simulink model "NMPC_MD_gaslift"  (R2023a)
settings: Solver=ode15s  StartTime=0.0  StopTime=par.simulation_time  FixedStep=par.sample_time  RelTol=1e-3
values from neighbouring files (symbols this model uses):
  par = function_parameters_NMPC_MD_gaslift    [main_NMPC_MD_gaslift.m]
  u0 = [par.Qginj0; par.pres]    [main_NMPC_MD_gaslift.m]
  x0 = [par.mg0; par.ml0; 0]    [main_NMPC_MD_gaslift.m]
libraries: sharedTrackingLibrary x1, mpclib x1
settings Model: Creator=aslik  LastModifiedBy=aslik
settings DataIOCC: ReturnWorkspaceOutputs=off  DatasetSignalFormat=timetable

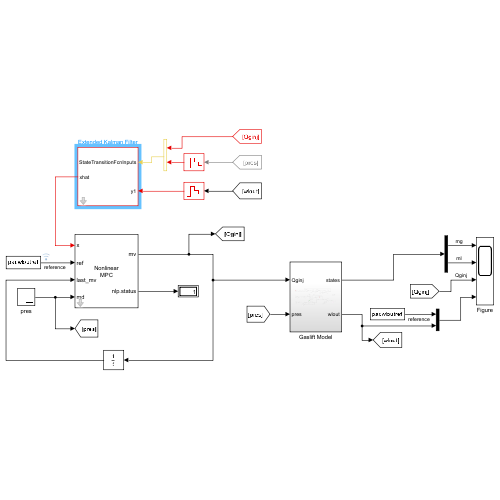
[thumbnail: Simulink's stored preview of the top-level diagram]
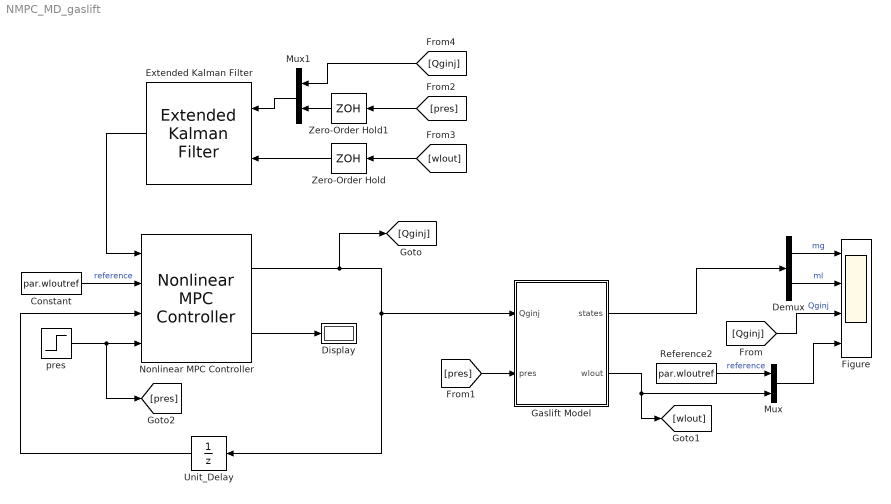
== system NMPC_MD_gaslift ==
  Constant : Constant  Value=par.wloutref  OutDataTypeStr=double  SampleTime=0
  Demux : Demux  Outputs=2
  Display : Display
  Extended Kalman Filter : sharedTrackingLibrary/Extended Kalman Filter  StateTransitionFcn=function_state_discrete_MD_gaslift  HasStateTransitionJacobianFcn=off  HasAdditiveProcessNoise=Additive  ProcessNoise=[2.213446776634616e-09,-7.436473103160610e-07,0;-7.436473103160610e-07,2.499957800870366e-04,0;0,0,0.002500000000000]  HasTimeVaryingProcessNoise=off  HasStateTransitionFcnExtraArgument=1  InitialState=x0  InitialStateCovariance=[2.213446776634616e-09,-7.436473103160610e-07,0;-7.436473103160610e-07,2.499957800870366e-04,0;0,0,0.002500000000000]  MeasurementFcn1=function_measurement_MD_gaslift  HasMeasurementJacobianFcn1=off  HasMeasurementEnablePort1=off  HasAdditiveMeasurementNoise1=Additive  MeasurementNoise1=1  HasTimeVaryingMeasurementNoise1=off  HasMeasurementFcnExtraArgument1=0  HasMeasurementWrapping1=off  MeasurementFcn2=myMeasurementFcn  HasMeasurementJacobianFcn2=off  HasMeasurementEnablePort2=off  HasAdditiveMeasurementNoise2=Additive  MeasurementNoise2=1  HasTimeVaryingMeasurementNoise2=off  HasMeasurementFcnExtraArgument2=0  HasMeasurementWrapping2=off  MeasurementFcn3=myMeasurementFcn  HasMeasurementJacobianFcn3=off  HasMeasurementEnablePort3=off  HasAdditiveMeasurementNoise3=Additive  MeasurementNoise3=1  HasTimeVaryingMeasurementNoise3=off  HasMeasurementFcnExtraArgument3=0  HasMeasurementWrapping3=off  MeasurementFcn4=myMeasurementFcn  HasMeasurementJacobianFcn4=off  HasMeasurementEnablePort4=off  HasAdditiveMeasurementNoise4=Additive  MeasurementNoise4=1  HasTimeVaryingMeasurementNoise4=off  HasMeasurementFcnExtraArgument4=0  HasMeasurementWrapping4=off  MeasurementFcn5=myMeasurementFcn  HasMeasurementJacobianFcn5=off  HasMeasurementEnablePort5=off  HasAdditiveMeasurementNoise5=Additive  MeasurementNoise5=1  HasTimeVaryingMeasurementNoise5=off  HasMeasurementFcnExtraArgument5=0  HasMeasurementWrapping5=off  EnableMultirate=off  StateTransitionFcnSampleTime=1  MeasurementFcn1SampleTime=1  MeasurementFcn2SampleTime=1  MeasurementFcn3SampleTime=1  MeasurementFcn4SampleTime=1  MeasurementFcn5SampleTime=1  UseCurrentEstimator=on  OutputStateCovariance=off  DataType=double  SampleTime=par.sample_time  NumberOfMeasurements=1
  Figure : Scope  NumInputPorts=4
  Gaslift Model : Subsystem  Description=|
      | The simple gas lift model consists of two states, gas accumulation (kg) and liquid accumulation. 
      | Gas inflow rate is the manipulated variable and the liquid outflow rate is the control variable.
      | Well inlet pressure is the measured disturbance.
  Mux : Mux  Inputs=2
  Mux1 : Mux  Inputs=2
  Nonlinear MPC Controller : mpclib/Nonlinear MPC Controller  SCDEnableBlockLinearizationSpecification=on  nlmpcobj=nlobj  UseObjectTs=on  UseMEX=off  md_enabled=on  mvtarget_enabled=off  param_enabled=off  cost_enabled=off  mvseq_enabled=off  stateseq_enabled=off  ovseq_enabled=off  slack_enabled=off  status_enabled=on  ov_min=off  ov_max=off  mv_min=off  mv_max=off  mvrate_min=off  mvrate_max=off  state_min=off  state_max=off  ov_weight=off  mv_weight=off  mvrate_weight=off  ecr_weight=off  nlp_initialize=off
  Reference2 : Constant  Value=par.wloutref  SampleTime=0
  Unit_Delay : UnitDelay  InitialCondition=u0(1)  SampleTime=-1  HasFrameUpgradeWarning=on
  Zero-Order Hold : ZeroOrderHold  SampleTime=par.sample_time
  Zero-Order Hold1 : ZeroOrderHold  SampleTime=par.sample_time
  pres : Step  Time=20  Before=par.pres  After=par.pres_final  SampleTime=0
  wires:
  [Qginj] -> Figure/3  "Qginj"
  Extended Kalman Filter/1 -> Nonlinear MPC Controller/1
  Gaslift Model/1(states) -> Demux/1
  Constant/1 -> Nonlinear MPC Controller/2  "reference"
  [Qginj] -> Mux1/1
  Unit_Delay/1 -> Nonlinear MPC Controller/3
  Demux/1 -> Figure/1  "mg"
  Nonlinear MPC Controller/1 -> Gaslift Model/1(Qginj), Unit_Delay/1, [Qginj]
  Nonlinear MPC Controller/2 -> Display/1
  Demux/2 -> Figure/2  "ml"
  pres/1 -> [pres], Nonlinear MPC Controller/4
  [pres] -> Gaslift Model/2(pres)
  Reference2/1 -> Mux/1  "reference"
  Gaslift Model/2(wlout) -> [wlout], Mux/2
  Mux/1 -> Figure/4
  Zero-Order Hold1/1 -> Mux1/2
  Mux1/1 -> Extended Kalman Filter/1
  [pres] -> Zero-Order Hold1/1
  [wlout] -> Zero-Order Hold/1
  Zero-Order Hold/1 -> Extended Kalman Filter/2

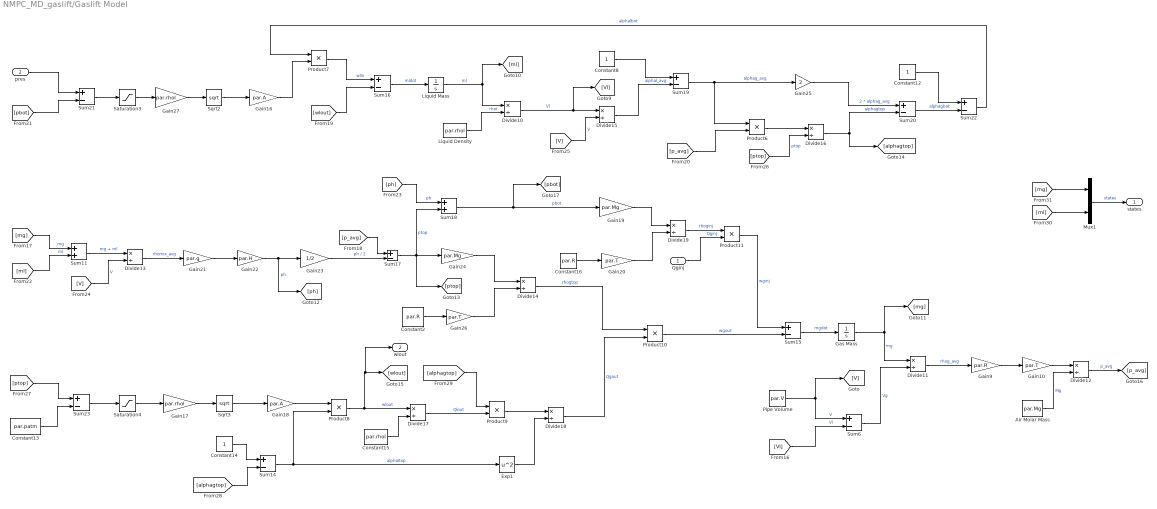
== system NMPC_MD_gaslift/Gaslift Model ==
  Qginj : Inport
  pres : Inport  Port=2
  Air Molar Mass : Constant  Value=par.Mg  OutDataTypeStr=double
  Constant12 : Constant  OutDataTypeStr=double
  Constant13 : Constant  Value=par.patm  OutDataTypeStr=double
  Constant14 : Constant  OutDataTypeStr=double
  Constant15 : Constant  Value=par.rhol  OutDataTypeStr=double
  Constant16 : Constant  Value=par.R  OutDataTypeStr=double
  Constant2 : Constant  Value=par.R  OutDataTypeStr=double
  Constant8 : Constant  OutDataTypeStr=double
  Divide{10..19} (10 alike) : Product  Inputs=*/
  Exp1 : Math  Operator=square
  Gain10 : Gain  Gain=par.T
  Gain16 : Gain  Gain=par.A
  Gain17 : Gain  Gain=par.rhol
  Gain18 : Gain  Gain=par.A
  Gain19 : Gain  Gain=par.Mg
  Gain20 : Gain  Gain=par.T
  Gain21 : Gain  Gain=par.g
  Gain22 : Gain  Gain=par.H
  Gain23 : Gain  Gain=1/2
  Gain24 : Gain  Gain=par.Mg
  Gain25 : Gain  Gain=2
  Gain26 : Gain  Gain=par.T
  Gain27 : Gain  Gain=par.rhol
  Gain9 : Gain  Gain=par.R
  "Gas Mass " : Integrator  InitialCondition=x0(1)  LowerSaturationLimit=0  ContinuousStateAttributes='mg'
  Liquid Density : Constant  Value=par.rhol  OutDataTypeStr=double
  Liquid Mass : Integrator  InitialCondition=x0(2)  LowerSaturationLimit=0  ContinuousStateAttributes='ml'
  Mux1 : Mux  Inputs=2
  Pipe Volume : Constant  Value=par.V  OutDataTypeStr=double
  Product{6..11} (6 alike) : Product
  Saturation3 : Saturate  UpperLimit=inf  LowerLimit=0
  Saturation4 : Saturate  UpperLimit=inf  LowerLimit=0
  Sqrt2 : Sqrt
  Sqrt3 : Sqrt
  Sum11 : Sum
  Sum{6,14..17,19..23} (10 alike) : Sum  Inputs=+-
  Sum18 : Sum
  states : Outport
  wlout : Outport  Port=2
  wires:
  [p_avg] -> Sum17/1
  Divide15/1 -> Sum19/2  "alphal_avg"
  Constant16/1 -> Gain20/1
  Divide17/1 -> Product9/2  "Qlout"
  [ptop] -> Divide16/2  "ptop"
  [ml] -> Mux1/2
  [wlout] -> Sum16/2
  Sum6/1 -> Divide11/2  "Vg"
  Saturation4/1 -> Gain17/1
  [alphagtop] -> Sum14/2
  Sum20/1 -> Sum22/2  "alphagbot"
  Divide19/1 -> Product11/1  "rhoginj"
  Sum18/1 -> [pbot], Gain19/1  "pbot"
  Sum22/1 -> Product7/1  "alphalbot"
  Pipe Volume/1 -> [V], Sum6/1  "V"
  [p_avg] -> Product6/2
  Divide10/1 -> Divide15/1, [Vl]  "Vl"
  Divide12/1 -> [p_avg]  "p_avg"
  [ml] -> Sum11/2  "ml"
  Sum17/1 -> Gain24/1, Sum18/2, [ptop]  "ptop"
  Gain19/1 -> Divide19/1
  Sum21/1 -> Saturation3/1
  Gain22/1 -> [ph], Gain23/1  "ph"
  Sqrt2/1 -> Gain16/1
  Product7/1 -> Sum16/1  "wlin"
  Product8/1 -> wlout/1, [wlout], Divide17/1  "wlout"
  [Vl] -> Sum6/2  "Vl"
  Gain23/1 -> Sum17/2  "ph / 2"
  Divide13/1 -> Gain21/1  "rhomix_avg"
  Constant12/1 -> Sum22/1
  Gain21/1 -> Gain22/1
  Sum23/1 -> Saturation4/1
  Gain17/1 -> Sqrt3/1
  Sum19/1 -> Product6/1, Gain25/1  "alphag_avg"
  [ph] -> Sum18/1  "ph"
  Qginj/1 -> Product11/2  "Qginj"
  [alphagtop] -> Product9/1
  Gain24/1 -> Divide14/1
  [ptop] -> Sum23/1
  Divide16/1 -> [alphagtop], Sum20/2  "alphagtop"
  Liquid Mass/1 -> [ml], Divide10/1  "ml"
  Saturation3/1 -> Gain27/1
  Product6/1 -> Divide16/1
  Sqrt3/1 -> Gain18/1
  [V] -> Divide15/2  "V"
  Gain9/1 -> Gain10/1
  Mux1/1 -> states/1  "states"
  Gain27/1 -> Sqrt2/1
  Constant2/1 -> Gain26/1
  pres/1 -> Sum21/1
  [mg] -> Sum11/1  "mg"
  Gain25/1 -> Sum20/1  "2 * alphag_avg"
  Gain16/1 -> Product7/2
  Air Molar Mass/1 -> Divide12/2  "Mg"
  Divide14/1 -> Product10/1  "rhogtop"
  Gain20/1 -> Divide19/2
  Sum15/1 -> "Gas Mass "/1  "mgdot"
  Divide11/1 -> Gain9/1  "rhog_avg"
  Exp1/1 -> Divide18/2
  Sum16/1 -> Liquid Mass/1  "mldot"
  "Gas Mass "/1 -> [mg], Divide11/1  "mg"
  [V] -> Divide13/2  "V"
  Product10/1 -> Sum15/2  "wgout"
  Constant8/1 -> Sum19/1
  Sum11/1 -> Divide13/1  "mg + ml"
  Gain18/1 -> Product8/1
  Divide18/1 -> Product10/2  "Qgout"
  Constant14/1 -> Sum14/1
  Product11/1 -> Sum15/1  "wginj"
  Liquid Density/1 -> Divide10/2  "rhol"
  [mg] -> Mux1/1
  Product9/1 -> Divide18/1
  [pbot] -> Sum21/2
  Sum14/1 -> Product8/2, Exp1/1  "alphaltop"
  Constant13/1 -> Sum23/2
  Gain26/1 -> Divide14/2
  Constant15/1 -> Divide17/2
  Gain10/1 -> Divide12/1
